simulink model "sf_msg_acknowledge"  (R2017b)
settings: Solver=ode45  StartTime=0.0  StopTime=20.0  RelTol=1e-3  EnableMultiTasking=on
settings Model: Creator=The MathWorks, Inc.  LastModifiedBy=The MathWorks, Inc.
settings DataIOCC: LimitDataPoints=on
settings OptimizationCC: LifeSpan=inf
settings DebuggingCC: AllowSymbolicDim=off  SFUnexpectedBacktrackingDiag=warning  SFNoUnconditionalDefaultTransitionDiag=warning  SFExecutionAtInitializationDiag=none
settings HardwareCC: ProdBitPerPointer=32  ProdBitPerSizeT=32  ProdBitPerPtrDiffT=32  ProdLargestAtomicFloat=None  ProdIntDivRoundTo=Undefined  ProdEndianess=Unspecified  ProdWordSize=32  ProdHWDeviceType=32-bit Generic
settings ModelReferenceCC: PropagateSignalLabelsOutOfModel=off
settings CodeAppCC: StateflowObjectComments=on
settings GRTTargetCC: TargetLangStandard=C89/C90 (ANSI)
settings ConfigComp: CovMetricSettings=dw  CovHtmlReporting=on  CovSaveCumulativeToWorkspaceVar=on  CovSaveSingleToWorkspaceVar=on  CovExternalEMLEnable=off

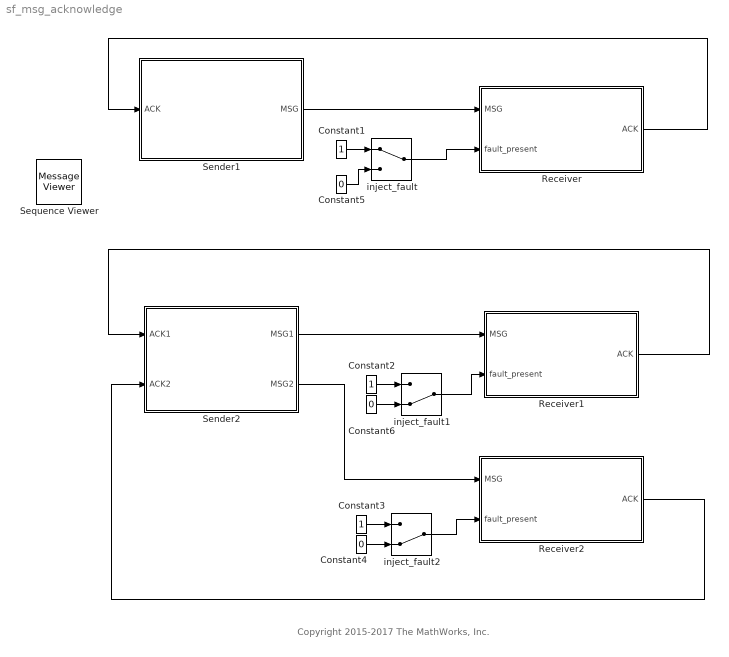
== system sf_msg_acknowledge ==
  note: Copyright 2015-2017 The MathWorks, Inc.
  Constant1 : Constant
  Constant2 : Constant
  Constant3 : Constant
  Constant4 : Constant  Value=0
  Constant5 : Constant  Value=0
  Constant6 : Constant  Value=0
  Receiver : Stateflow chart  TreatAsAtomicUnit=on
  Receiver1 : Stateflow chart  TreatAsAtomicUnit=on
  Receiver2 : Stateflow chart  TreatAsAtomicUnit=on
  Sender1 : Stateflow chart  TreatAsAtomicUnit=on
  Sender2 : Stateflow chart  TreatAsAtomicUnit=on
  Sequence Viewer : MessageViewer
  inject_fault : ManualSwitch
  inject_fault1 : ManualSwitch  CurrentSetting=0
  inject_fault2 : ManualSwitch  CurrentSetting=0
  wires:
  Sender1/1(MSG) -> Receiver/1(MSG)
  Receiver/1(ACK) -> Sender1/1(ACK)
  inject_fault/1 -> Receiver/2(fault_present)
  Constant5/1 -> inject_fault/2
  Constant1/1 -> inject_fault/1
  Sender2/1(MSG1) -> Receiver1/1(MSG)
  inject_fault1/1 -> Receiver1/2(fault_present)
  Constant6/1 -> inject_fault1/2
  Constant2/1 -> inject_fault1/1
  Constant4/1 -> inject_fault2/2
  Constant3/1 -> inject_fault2/1
  inject_fault2/1 -> Receiver2/2(fault_present)
  Sender2/2(MSG2) -> Receiver2/1(MSG)
  Receiver1/1(ACK) -> Sender2/1(ACK1)
  Receiver2/1(ACK) -> Sender2/2(ACK2)

== stateflow chart sf_msg_acknowledge/Receiver ==
  state Idle
  state Processing
  state SendAcknowledgement
    entry:
    ACK.data = 1;
    send(ACK);
  (default) -> Idle
  Processing -> Idle [order 2] : [fault_present]
  Idle -> Processing : MSG
  Processing -> SendAcknowledgement [order 1] : after(5,sec)
  data: MSG input; ACK output; fault_present input

== stateflow chart sf_msg_acknowledge/Receiver1 ==
  state Idle
  state Processing
  state SendAcknowledgement
    entry:
    ACK.data = 1;
    send(ACK);
  (default) -> Idle
  Processing -> Idle [order 2] : [fault_present]
  Idle -> Processing : MSG
  Processing -> SendAcknowledgement [order 1] : after(5,sec)
  data: MSG input; ACK output; fault_present input

== stateflow chart sf_msg_acknowledge/Sender1 ==
  state Idle
  state SendMessageAndWait
    entry:
    MSG.data=1;
    send(MSG);
  state TimedOut
  state Done
  (default) -> Idle
  Idle -> SendMessageAndWait
  SendMessageAndWait -> TimedOut [order 2] : after(10,sec)
  SendMessageAndWait -> Done [order 1] : ACK
  data: ACK input; MSG output

== stateflow chart sf_msg_acknowledge/Receiver2 ==
  state Idle
  state Processing
  state SendAcknowledgement
    entry:
    ACK.data = 1;
    send(ACK);
  (default) -> Idle
  Processing -> Idle [order 2] : [fault_present]
  Idle -> Processing : MSG
  Processing -> SendAcknowledgement [order 1] : after(10,sec)
  data: MSG input; ACK output; fault_present input

== stateflow chart sf_msg_acknowledge/Sender2 ==
  state Idle
  state SendMessage
    entry:
    MSG1.data=1;
    send(MSG1);
    MSG2.data=1;
    send(MSG2);
  state WaitForAcknowledgements
    entry:
    ackCount =0;
    on ACK1: ackCount = ackCount + 1;
    on ACK2: ackCount = ackCount + 1;
  state TimedOut
  state Done
  (default) -> Idle
  Idle -> SendMessage
  SendMessage -> WaitForAcknowledgements
  WaitForAcknowledgements -> TimedOut [order 1] : after(15,sec)
  WaitForAcknowledgements -> Done [order 2] : [ackCount==2]
  data: MSG1 output; MSG2 output; ACK1 input; ACK2 input; ackCount local
